simulink model "multipath_fading1"  (Simulink 5.0)
settings: Solver=ode45  StartTime=0.0  StopTime=1  RelTol=1e-3
undefined symbols (not defined in the file): get, p, y
libraries: dspmathops x40, dspstat3 x1, simulink x1, dspsnks4 x1
(part 1 of 2)
settings Model: LastModifiedBy=Daiming Qu  LimitDataPoints=off  SignalLoggingName=logsout  RTWOptions="-aEnforceIntegerDowncast=1 -aExtMode=0 -aExtModeTesting=0 -aFoldNonRolledExpr=1 -aForceParamTrailComments=0 -aGenerateComments=1 -aGenerateReport=0 -aIgnoreCustomStorageClasses=1 -aIncDataTypeInIds=0 -aIncHierarchyInIds=0 -aInlineInvariantSignals=0 -aInlinedPrmAccess=\"Literals\" -aLocalBlockOutputs=1 -aLogVarNameModifier=\"rt_\" -aMaxRTWIdLen=31 -aPrefixModelToSubsysFcnNames=1 -aRTWVerbose=1 -aRollThreshold=5 -aShowEliminatedStatements=0"

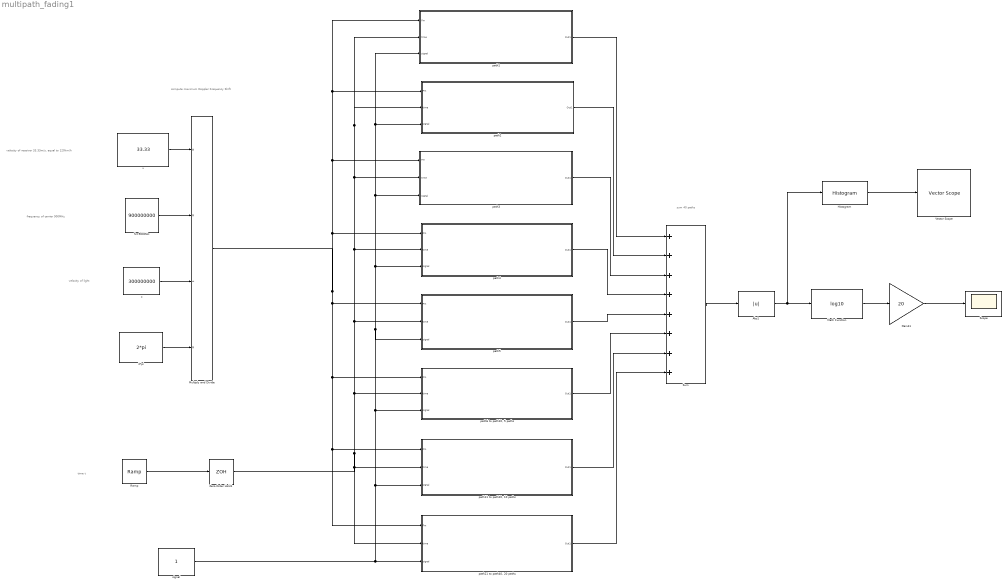
== system multipath_fading1 ==
  note: compute maximum
      | Doppler Frequency Shift
  note: velocity
      |  of light
  note: frequency of carrier
      |  900MHz
  note: velocity of receiver
      | 33.33m/s,
      | equal to 120km/h
  note: sum 40 paths
  note: time t
  2*pi : Constant  Value=2*pi
  Abs1 : Abs
  Gain41 : Gain  Gain=20
  Histogram : dspstat3/Histogram  umin=0  umax=20  nbins=1000  normalized=off  run=on  reset=off  trigtype=Non-zero sample
  Math Function : Math  Operator=log10
  Multiply and Divide : Product  Inputs=**/*  OutScaling=2^-10
  Ramp : simulink/Sources/Ramp  slope=1  start=0  X0=0
  Scope : Scope
      settings: TimeRange=0.06705882352941177  YMax=11  SaveName=ScopeData4
  Sum : Sum  Inputs=++++++++  OutScaling=2^-10
  Vector Scope : dspsnks4/Vector Scope  ScopeProperties=off  Domain=User-defined  HorizSpan=1  DisplayProperties=off  AxisGrid=on  Memory=off  FrameNumber=on  AxisLegend=off  AxisZoom=off  OpenScopeAtSimStart=on  OpenScopeImmediately=off  FigPos=get(0,'defaultfigureposition')  AxisProperties=on  XUnits=Hertz  XRange=[0...Fs/2]  InheritXIncr=on  XIncr=1  XLabel=y  YUnits=dB  YLabel=p(y)  LineProperties=off  LineColors=[0 0 0]
      settings: YMin=0  YMax=700
  Zero-Order Hold1 : ZeroOrderHold  SampleTime=0.00001
  c : Constant  Value=300000000
  fc=900MHz : Constant  Value=900000000
  path1 : Subsystem
  "path11 to path20, 10 paths" : Subsystem
  path2 : Subsystem
  "path21 to path40, 20 paths" : Subsystem
  path3 : Subsystem
  path4 : Subsystem
  path5 : Subsystem
  "path6 to path10, 5 paths" : Subsystem
  signal : Constant
  v : Constant  Value=33.33
  wires:
  fc=900MHz/1 -> Multiply and Divide/2
  c/1 -> Multiply and Divide/3
  v/1 -> Multiply and Divide/1
  Math Function/1 -> Gain41/1
  2*pi/1 -> Multiply and Divide/4
  Gain41/1 -> Scope/1
  Multiply and Divide/1 -> path1/1(Fm), path2/1(Fm), path3/1(Fm), path4/1(Fm), "path6 to path10, 5 paths"/1(Fm), "path21 to path40, 20 paths"/1(Fm), "path11 to path20, 10 paths"/1(Fm), path5/1(Fm)
  path1/1(Out1) -> Sum/1
  "path21 to path40, 20 paths"/1(Out1) -> Sum/8
  "path11 to path20, 10 paths"/1(Out1) -> Sum/7
  "path6 to path10, 5 paths"/1(Out1) -> Sum/6
  Ramp/1 -> Zero-Order Hold1/1
  Zero-Order Hold1/1 -> "path6 to path10, 5 paths"/2(time), path1/2(time), path2/2(time), path3/2(time), path4/2(time), path5/2(time), "path21 to path40, 20 paths"/2(time), "path11 to path20, 10 paths"/2(time)
  Histogram/1 -> Vector Scope/1
  Sum/1 -> Abs1/1
  Abs1/1 -> Histogram/1, Math Function/1
  path2/1(Out1) -> Sum/2
  path3/1(Out1) -> Sum/3
  path4/1(Out1) -> Sum/4
  path5/1(Out1) -> Sum/5
  signal/1 -> "path21 to path40, 20 paths"/3(signal), "path11 to path20, 10 paths"/3(signal), "path6 to path10, 5 paths"/3(signal), path5/3(signal), path4/3(signal), path3/3(signal), path2/3(signal), path1/3(signal)

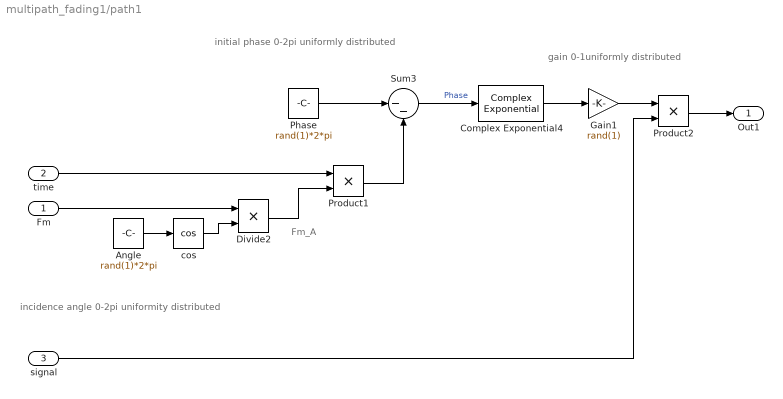
== system multipath_fading1/path1 ==
  note: initial phase
      | 0-2pi
      | uniformly
      | distributed
  note: incidence angle
      | 0-2pi
      | uniformity
      | distributed
  note: gain
      | 0-1uniformly distributed
  note: Fm_A
  Fm : Inport
  time : Inport  Port=2
  signal : Inport  Port=3
  Angle : Constant  Value=rand(1)*2*pi
  Complex Exponential4 : dspmathops/Complex Exponential
  Divide2 : Product  Inputs=**  OutScaling=2^-10
  Gain1 : Gain  Gain=rand(1)
  Phase : Constant  Value=rand(1)*2*pi
  Product1 : Product  RndMeth=Zero
  Product2 : Product  RndMeth=Zero
  Sum3 : Sum  Inputs=|--
  cos : Trigonometry  Operator=cos
  Out1 : Outport
  wires:
  Phase/1 -> Sum3/1
  Complex Exponential4/1 -> Gain1/1
  Sum3/1 -> Complex Exponential4/1  "Phase"
  Angle/1 -> cos/1
  Fm/1 -> Divide2/1
  cos/1 -> Divide2/2
  time/1 -> Product1/1
  Divide2/1 -> Product1/2
  Product1/1 -> Sum3/2
  Gain1/1 -> Product2/1
  Product2/1 -> Out1/1
  signal/1 -> Product2/2

== system multipath_fading1/path11 to path20, 10 paths ==
  Fm : Inport
  time : Inport  Port=2
  signal : Inport  Port=3
  Add : Sum  OutScaling=2^-10
  "path11 to path15, 5 paths" : Subsystem
  "path16 to path20, 5 paths" : Subsystem
  Out1 : Outport
  wires:
  Add/1 -> Out1/1
  Fm/1 -> "path11 to path15, 5 paths"/1(Fm), "path16 to path20, 5 paths"/1(Fm)
  "path11 to path15, 5 paths"/1(Out1) -> Add/1
  time/1 -> "path11 to path15, 5 paths"/2(Time), "path16 to path20, 5 paths"/2(Time)
  "path16 to path20, 5 paths"/1(Out1) -> Add/2
  signal/1 -> "path11 to path15, 5 paths"/3(signal), "path16 to path20, 5 paths"/3(signal)

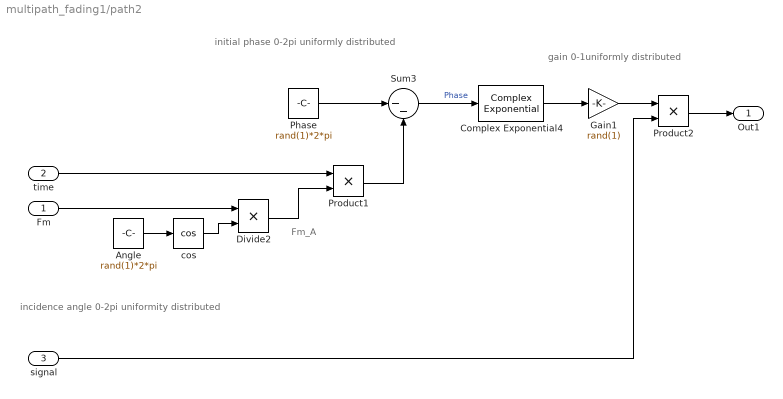
== system multipath_fading1/path2 ==
  note: initial phase
      | 0-2pi
      | uniformly
      | distributed
  note: incidence angle
      | 0-2pi
      | uniformity
      | distributed
  note: gain
      | 0-1uniformly distributed
  note: Fm_A
  Fm : Inport
  time : Inport  Port=2
  signal : Inport  Port=3
  Angle : Constant  Value=rand(1)*2*pi
  Complex Exponential4 : dspmathops/Complex Exponential
  Divide2 : Product  Inputs=**  OutScaling=2^-10
  Gain1 : Gain  Gain=rand(1)
  Phase : Constant  Value=rand(1)*2*pi
  Product1 : Product  RndMeth=Zero
  Product2 : Product  RndMeth=Zero
  Sum3 : Sum  Inputs=|--
  cos : Trigonometry  Operator=cos
  Out1 : Outport
  wires:
  Phase/1 -> Sum3/1
  Complex Exponential4/1 -> Gain1/1
  Sum3/1 -> Complex Exponential4/1  "Phase"
  Angle/1 -> cos/1
  Fm/1 -> Divide2/1
  cos/1 -> Divide2/2
  time/1 -> Product1/1
  Divide2/1 -> Product1/2
  Product1/1 -> Sum3/2
  Gain1/1 -> Product2/1
  Product2/1 -> Out1/1
  signal/1 -> Product2/2

== system multipath_fading1/path21 to path40, 20 paths ==
  Fm : Inport
  time : Inport  Port=2
  signal : Inport  Port=3
  Add : Sum  OutScaling=2^-10
  "path21 to path30, 10 paths" : Subsystem
  "path31 to path40, 10 paths" : Subsystem
  Out1 : Outport
  wires:
  "path31 to path40, 10 paths"/1(Out1) -> Add/2
  time/1 -> "path21 to path30, 10 paths"/2(time), "path31 to path40, 10 paths"/2(time)
  "path21 to path30, 10 paths"/1(Out1) -> Add/1
  Fm/1 -> "path21 to path30, 10 paths"/1(Fm), "path31 to path40, 10 paths"/1(Fm)
  Add/1 -> Out1/1
  signal/1 -> "path21 to path30, 10 paths"/3(signal), "path31 to path40, 10 paths"/3(signal)

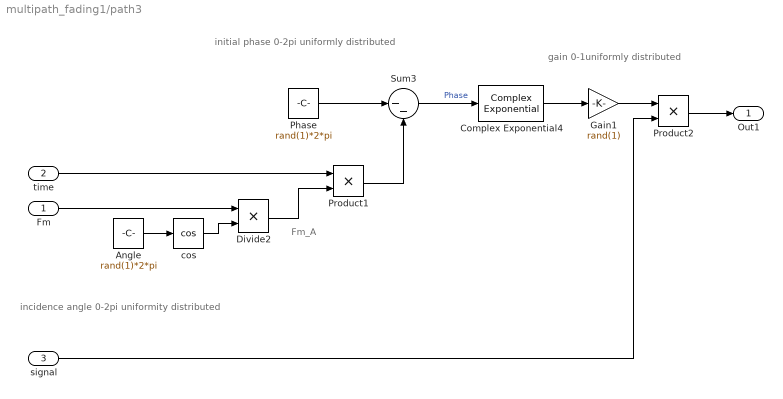
== system multipath_fading1/path3 ==
  note: initial phase
      | 0-2pi
      | uniformly
      | distributed
  note: incidence angle
      | 0-2pi
      | uniformity
      | distributed
  note: gain
      | 0-1uniformly distributed
  note: Fm_A
  Fm : Inport
  time : Inport  Port=2
  signal : Inport  Port=3
  Angle : Constant  Value=rand(1)*2*pi
  Complex Exponential4 : dspmathops/Complex Exponential
  Divide2 : Product  Inputs=**  OutScaling=2^-10
  Gain1 : Gain  Gain=rand(1)
  Phase : Constant  Value=rand(1)*2*pi
  Product1 : Product  RndMeth=Zero
  Product2 : Product  RndMeth=Zero
  Sum3 : Sum  Inputs=|--
  cos : Trigonometry  Operator=cos
  Out1 : Outport
  wires:
  Phase/1 -> Sum3/1
  Complex Exponential4/1 -> Gain1/1
  Sum3/1 -> Complex Exponential4/1  "Phase"
  Angle/1 -> cos/1
  Fm/1 -> Divide2/1
  cos/1 -> Divide2/2
  time/1 -> Product1/1
  Divide2/1 -> Product1/2
  Product1/1 -> Sum3/2
  Gain1/1 -> Product2/1
  Product2/1 -> Out1/1
  signal/1 -> Product2/2

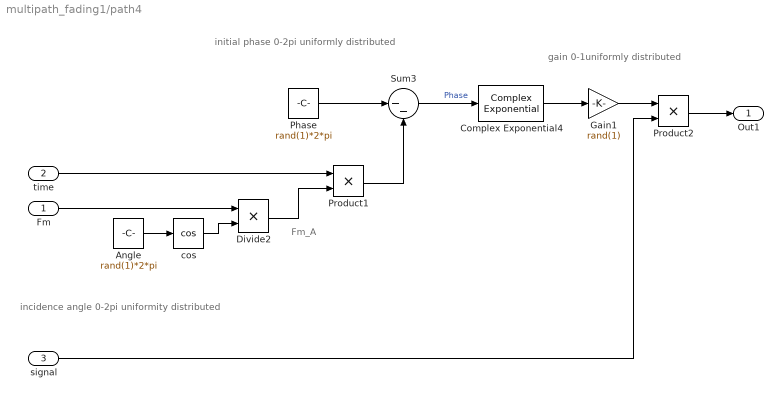
== system multipath_fading1/path4 ==
  note: initial phase
      | 0-2pi
      | uniformly
      | distributed
  note: incidence angle
      | 0-2pi
      | uniformity
      | distributed
  note: gain
      | 0-1uniformly distributed
  note: Fm_A
  Fm : Inport
  time : Inport  Port=2
  signal : Inport  Port=3
  Angle : Constant  Value=rand(1)*2*pi
  Complex Exponential4 : dspmathops/Complex Exponential
  Divide2 : Product  Inputs=**  OutScaling=2^-10
  Gain1 : Gain  Gain=rand(1)
  Phase : Constant  Value=rand(1)*2*pi
  Product1 : Product  RndMeth=Zero
  Product2 : Product  RndMeth=Zero
  Sum3 : Sum  Inputs=|--
  cos : Trigonometry  Operator=cos
  Out1 : Outport
  wires:
  Phase/1 -> Sum3/1
  Complex Exponential4/1 -> Gain1/1
  Sum3/1 -> Complex Exponential4/1  "Phase"
  Angle/1 -> cos/1
  Fm/1 -> Divide2/1
  cos/1 -> Divide2/2
  time/1 -> Product1/1
  Divide2/1 -> Product1/2
  Product1/1 -> Sum3/2
  Gain1/1 -> Product2/1
  Product2/1 -> Out1/1
  signal/1 -> Product2/2

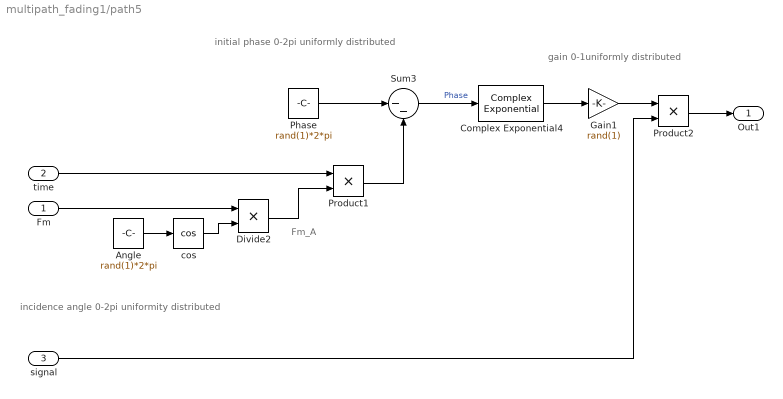
== system multipath_fading1/path5 ==
  note: initial phase
      | 0-2pi
      | uniformly
      | distributed
  note: incidence angle
      | 0-2pi
      | uniformity
      | distributed
  note: gain
      | 0-1uniformly distributed
  note: Fm_A
  Fm : Inport
  time : Inport  Port=2
  signal : Inport  Port=3
  Angle : Constant  Value=rand(1)*2*pi
  Complex Exponential4 : dspmathops/Complex Exponential
  Divide2 : Product  Inputs=**  OutScaling=2^-10
  Gain1 : Gain  Gain=rand(1)
  Phase : Constant  Value=rand(1)*2*pi
  Product1 : Product  RndMeth=Zero
  Product2 : Product  RndMeth=Zero
  Sum3 : Sum  Inputs=|--
  cos : Trigonometry  Operator=cos
  Out1 : Outport
  wires:
  Phase/1 -> Sum3/1
  Complex Exponential4/1 -> Gain1/1
  Sum3/1 -> Complex Exponential4/1  "Phase"
  Angle/1 -> cos/1
  Fm/1 -> Divide2/1
  cos/1 -> Divide2/2
  time/1 -> Product1/1
  Divide2/1 -> Product1/2
  Product1/1 -> Sum3/2
  Gain1/1 -> Product2/1
  Product2/1 -> Out1/1
  signal/1 -> Product2/2

== system multipath_fading1/path6 to path10, 5 paths ==
  Fm : Inport
  time : Inport  Port=2
  signal : Inport  Port=3
  Add : Sum  Inputs=+++++  OutScaling=2^-10
  path1 : Subsystem
  path6 : Subsystem
  path7 : Subsystem
  path8 : Subsystem
  path9 : Subsystem
  Out1 : Outport
  wires:
  Fm/1 -> path9/1(Fm), path1/1(Fm), path8/1(Fm), path7/1(Fm), path6/1(Fm)
  time/1 -> path6/2(time), path7/2(time), path8/2(time), path9/2(time), path1/2(time)
  Add/1 -> Out1/1
  path8/1(Out1) -> Add/3
  path9/1(Out1) -> Add/4
  path7/1(Out1) -> Add/2
  path6/1(Out1) -> Add/1
  path1/1(Out1) -> Add/5
  signal/1 -> path6/3(signal), path7/3(signal), path8/3(signal), path9/3(signal), path1/3(signal)

== system multipath_fading1/path11 to path20, 10 paths/path11 to path15, 5 paths ==
  Fm : Inport
  Time : Inport  Port=2
  signal : Inport  Port=3
  Add : Sum  Inputs=+++++  OutScaling=2^-10
  path11 : Subsystem
  path12 : Subsystem
  path13 : Subsystem
  path14 : Subsystem
  path15 : Subsystem
  Out1 : Outport
  wires:
  Fm/1 -> path14/1(Fm), path15/1(Fm), path13/1(Fm), path12/1(Fm), path11/1(Fm)
  Time/1 -> path11/2(time), path12/2(time), path13/2(time), path14/2(time), path15/2(time)
  Add/1 -> Out1/1
  path13/1(Out1) -> Add/3
  path14/1(Out1) -> Add/4
  path12/1(Out1) -> Add/2
  path11/1(Out1) -> Add/1
  path15/1(Out1) -> Add/5
  signal/1 -> path11/3(signal), path12/3(signal), path13/3(signal), path14/3(signal), path15/3(signal)

== system multipath_fading1/path11 to path20, 10 paths/path16 to path20, 5 paths ==
  Fm : Inport
  Time : Inport  Port=2
  signal : Inport  Port=3
  Add : Sum  Inputs=+++++  OutScaling=2^-10
  path16 : Subsystem
  path17 : Subsystem
  path18 : Subsystem
  path19 : Subsystem
  path20 : Subsystem
  Out1 : Outport
  wires:
  Fm/1 -> path19/1(Fm), path20/1(Fm), path18/1(Fm), path17/1(Fm), path16/1(Fm)
  Time/1 -> path16/2(time), path17/2(time), path18/2(time), path19/2(time), path20/2(time)
  Add/1 -> Out1/1
  path18/1(Out1) -> Add/3
  path19/1(Out1) -> Add/4
  path17/1(Out1) -> Add/2
  path16/1(Out1) -> Add/1
  path20/1(Out1) -> Add/5
  signal/1 -> path16/3(signal), path17/3(signal), path18/3(signal), path19/3(signal), path20/3(signal)

== system multipath_fading1/path21 to path40, 20 paths/path21 to path30, 10 paths ==
  Fm : Inport
  time : Inport  Port=2
  signal : Inport  Port=3
  Add : Sum  OutScaling=2^-10
  "path21 to path25, 5 paths" : Subsystem
  "path26 to path30, 5 paths" : Subsystem
  Out1 : Outport
  wires:
  Add/1 -> Out1/1
  Fm/1 -> "path21 to path25, 5 paths"/1(Fm), "path26 to path30, 5 paths"/1(Fm)
  "path21 to path25, 5 paths"/1(Out1) -> Add/1
  time/1 -> "path21 to path25, 5 paths"/2(Time), "path26 to path30, 5 paths"/2(Time)
  "path26 to path30, 5 paths"/1(Out1) -> Add/2
  signal/1 -> "path21 to path25, 5 paths"/3(signal), "path26 to path30, 5 paths"/3(signal)

== system multipath_fading1/path21 to path40, 20 paths/path31 to path40, 10 paths ==
  Fm : Inport
  time : Inport  Port=2
  signal : Inport  Port=3
  Add : Sum  OutScaling=2^-10
  "path31 to path35, 5 paths" : Subsystem
  "path36 to path40, 5 paths" : Subsystem
  Out1 : Outport
  wires:
  Add/1 -> Out1/1
  Fm/1 -> "path31 to path35, 5 paths"/1(Fm), "path36 to path40, 5 paths"/1(Fm)
  "path31 to path35, 5 paths"/1(Out1) -> Add/1
  time/1 -> "path31 to path35, 5 paths"/2(Time), "path36 to path40, 5 paths"/2(Time)
  "path36 to path40, 5 paths"/1(Out1) -> Add/2
  signal/1 -> "path31 to path35, 5 paths"/3(signal), "path36 to path40, 5 paths"/3(signal)

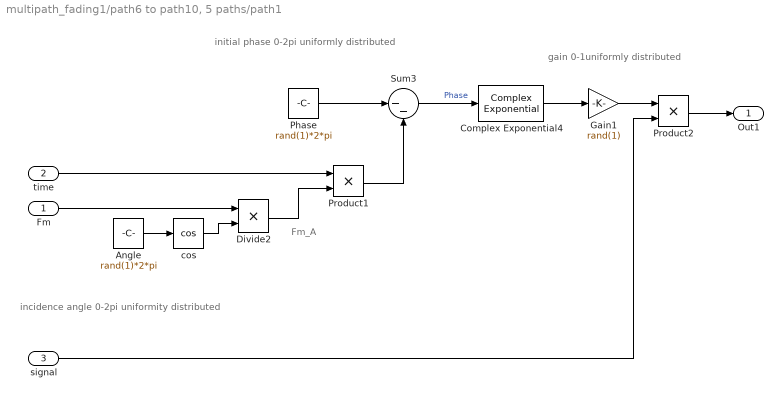
== system multipath_fading1/path6 to path10, 5 paths/path1 ==
  note: initial phase
      | 0-2pi
      | uniformly
      | distributed
  note: incidence angle
      | 0-2pi
      | uniformity
      | distributed
  note: gain
      | 0-1uniformly distributed
  note: Fm_A
  Fm : Inport
  time : Inport  Port=2
  signal : Inport  Port=3
  Angle : Constant  Value=rand(1)*2*pi
  Complex Exponential4 : dspmathops/Complex Exponential
  Divide2 : Product  Inputs=**  OutScaling=2^-10
  Gain1 : Gain  Gain=rand(1)
  Phase : Constant  Value=rand(1)*2*pi
  Product1 : Product  RndMeth=Zero
  Product2 : Product  RndMeth=Zero
  Sum3 : Sum  Inputs=|--
  cos : Trigonometry  Operator=cos
  Out1 : Outport
  wires:
  Phase/1 -> Sum3/1
  Complex Exponential4/1 -> Gain1/1
  Sum3/1 -> Complex Exponential4/1  "Phase"
  Angle/1 -> cos/1
  Fm/1 -> Divide2/1
  cos/1 -> Divide2/2
  time/1 -> Product1/1
  Divide2/1 -> Product1/2
  Product1/1 -> Sum3/2
  Gain1/1 -> Product2/1
  Product2/1 -> Out1/1
  signal/1 -> Product2/2

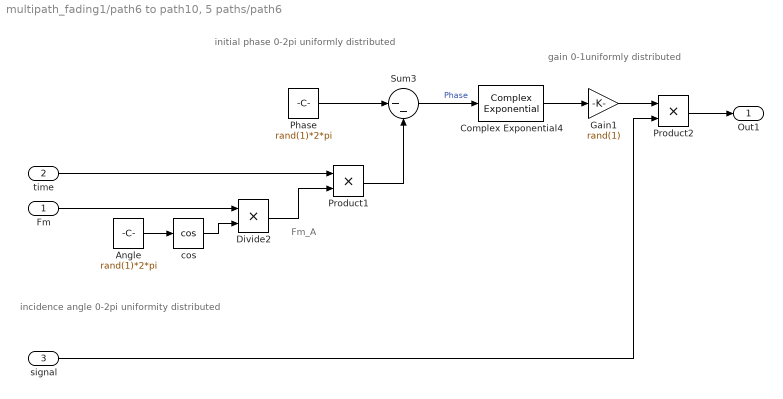
== system multipath_fading1/path6 to path10, 5 paths/path6 ==
  note: initial phase
      | 0-2pi
      | uniformly
      | distributed
  note: incidence angle
      | 0-2pi
      | uniformity
      | distributed
  note: gain
      | 0-1uniformly distributed
  note: Fm_A
  Fm : Inport
  time : Inport  Port=2
  signal : Inport  Port=3
  Angle : Constant  Value=rand(1)*2*pi
  Complex Exponential4 : dspmathops/Complex Exponential
  Divide2 : Product  Inputs=**  OutScaling=2^-10
  Gain1 : Gain  Gain=rand(1)
  Phase : Constant  Value=rand(1)*2*pi
  Product1 : Product  RndMeth=Zero
  Product2 : Product  RndMeth=Zero
  Sum3 : Sum  Inputs=|--
  cos : Trigonometry  Operator=cos
  Out1 : Outport
  wires:
  Phase/1 -> Sum3/1
  Complex Exponential4/1 -> Gain1/1
  Sum3/1 -> Complex Exponential4/1  "Phase"
  Angle/1 -> cos/1
  Fm/1 -> Divide2/1
  cos/1 -> Divide2/2
  time/1 -> Product1/1
  Divide2/1 -> Product1/2
  Product1/1 -> Sum3/2
  Gain1/1 -> Product2/1
  Product2/1 -> Out1/1
  signal/1 -> Product2/2

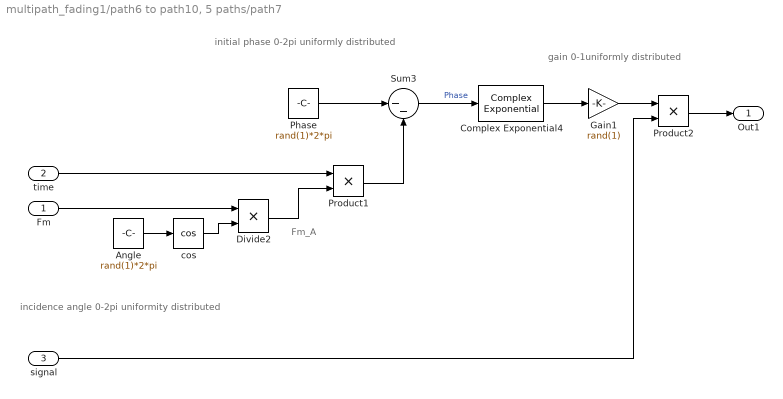
== system multipath_fading1/path6 to path10, 5 paths/path7 ==
  note: initial phase
      | 0-2pi
      | uniformly
      | distributed
  note: incidence angle
      | 0-2pi
      | uniformity
      | distributed
  note: gain
      | 0-1uniformly distributed
  note: Fm_A
  Fm : Inport
  time : Inport  Port=2
  signal : Inport  Port=3
  Angle : Constant  Value=rand(1)*2*pi
  Complex Exponential4 : dspmathops/Complex Exponential
  Divide2 : Product  Inputs=**  OutScaling=2^-10
  Gain1 : Gain  Gain=rand(1)
  Phase : Constant  Value=rand(1)*2*pi
  Product1 : Product  RndMeth=Zero
  Product2 : Product  RndMeth=Zero
  Sum3 : Sum  Inputs=|--
  cos : Trigonometry  Operator=cos
  Out1 : Outport
  wires:
  Phase/1 -> Sum3/1
  Complex Exponential4/1 -> Gain1/1
  Sum3/1 -> Complex Exponential4/1  "Phase"
  Angle/1 -> cos/1
  Fm/1 -> Divide2/1
  cos/1 -> Divide2/2
  time/1 -> Product1/1
  Divide2/1 -> Product1/2
  Product1/1 -> Sum3/2
  Gain1/1 -> Product2/1
  Product2/1 -> Out1/1
  signal/1 -> Product2/2

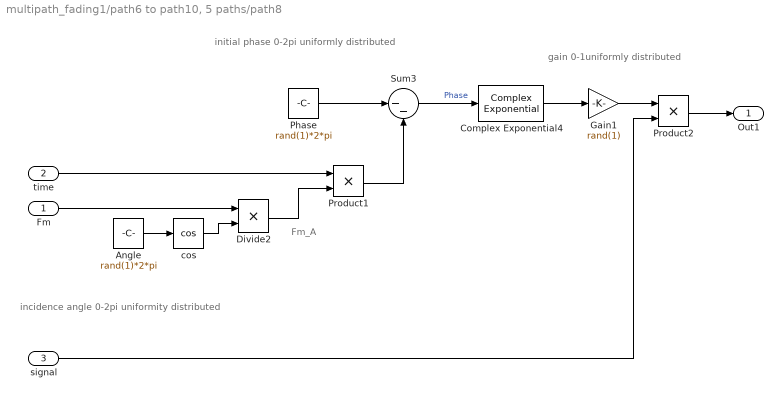
== system multipath_fading1/path6 to path10, 5 paths/path8 ==
  note: initial phase
      | 0-2pi
      | uniformly
      | distributed
  note: incidence angle
      | 0-2pi
      | uniformity
      | distributed
  note: gain
      | 0-1uniformly distributed
  note: Fm_A
  Fm : Inport
  time : Inport  Port=2
  signal : Inport  Port=3
  Angle : Constant  Value=rand(1)*2*pi
  Complex Exponential4 : dspmathops/Complex Exponential
  Divide2 : Product  Inputs=**  OutScaling=2^-10
  Gain1 : Gain  Gain=rand(1)
  Phase : Constant  Value=rand(1)*2*pi
  Product1 : Product  RndMeth=Zero
  Product2 : Product  RndMeth=Zero
  Sum3 : Sum  Inputs=|--
  cos : Trigonometry  Operator=cos
  Out1 : Outport
  wires:
  Phase/1 -> Sum3/1
  Complex Exponential4/1 -> Gain1/1
  Sum3/1 -> Complex Exponential4/1  "Phase"
  Angle/1 -> cos/1
  Fm/1 -> Divide2/1
  cos/1 -> Divide2/2
  time/1 -> Product1/1
  Divide2/1 -> Product1/2
  Product1/1 -> Sum3/2
  Gain1/1 -> Product2/1
  Product2/1 -> Out1/1
  signal/1 -> Product2/2

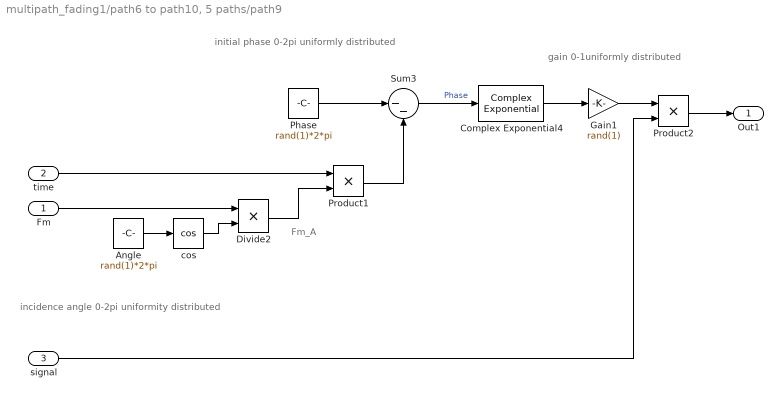
== system multipath_fading1/path6 to path10, 5 paths/path9 ==
  note: initial phase
      | 0-2pi
      | uniformly
      | distributed
  note: incidence angle
      | 0-2pi
      | uniformity
      | distributed
  note: gain
      | 0-1uniformly distributed
  note: Fm_A
  Fm : Inport
  time : Inport  Port=2
  signal : Inport  Port=3
  Angle : Constant  Value=rand(1)*2*pi
  Complex Exponential4 : dspmathops/Complex Exponential
  Divide2 : Product  Inputs=**  OutScaling=2^-10
  Gain1 : Gain  Gain=rand(1)
  Phase : Constant  Value=rand(1)*2*pi
  Product1 : Product  RndMeth=Zero
  Product2 : Product  RndMeth=Zero
  Sum3 : Sum  Inputs=|--
  cos : Trigonometry  Operator=cos
  Out1 : Outport
  wires:
  Phase/1 -> Sum3/1
  Complex Exponential4/1 -> Gain1/1
  Sum3/1 -> Complex Exponential4/1  "Phase"
  Angle/1 -> cos/1
  Fm/1 -> Divide2/1
  cos/1 -> Divide2/2
  time/1 -> Product1/1
  Divide2/1 -> Product1/2
  Product1/1 -> Sum3/2
  Gain1/1 -> Product2/1
  Product2/1 -> Out1/1
  signal/1 -> Product2/2

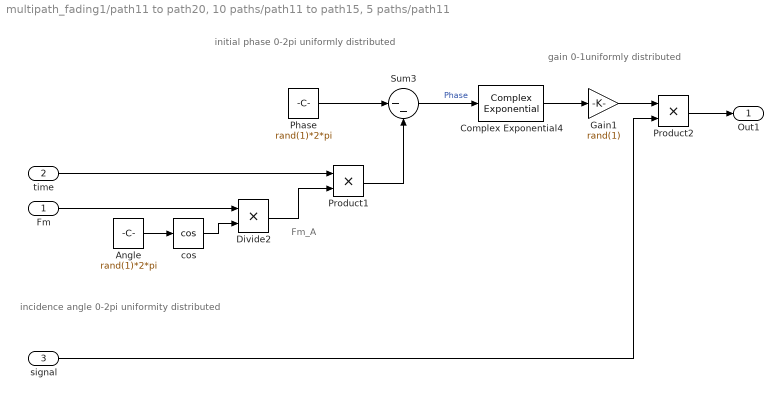
== system multipath_fading1/path11 to path20, 10 paths/path11 to path15, 5 paths/path11 ==
  note: initial phase
      | 0-2pi
      | uniformly
      | distributed
  note: incidence angle
      | 0-2pi
      | uniformity
      | distributed
  note: gain
      | 0-1uniformly distributed
  note: Fm_A
  Fm : Inport
  time : Inport  Port=2
  signal : Inport  Port=3
  Angle : Constant  Value=rand(1)*2*pi
  Complex Exponential4 : dspmathops/Complex Exponential
  Divide2 : Product  Inputs=**  OutScaling=2^-10
  Gain1 : Gain  Gain=rand(1)
  Phase : Constant  Value=rand(1)*2*pi
  Product1 : Product  RndMeth=Zero
  Product2 : Product  RndMeth=Zero
  Sum3 : Sum  Inputs=|--
  cos : Trigonometry  Operator=cos
  Out1 : Outport
  wires:
  Phase/1 -> Sum3/1
  Complex Exponential4/1 -> Gain1/1
  Sum3/1 -> Complex Exponential4/1  "Phase"
  Angle/1 -> cos/1
  Fm/1 -> Divide2/1
  cos/1 -> Divide2/2
  time/1 -> Product1/1
  Divide2/1 -> Product1/2
  Product1/1 -> Sum3/2
  Gain1/1 -> Product2/1
  Product2/1 -> Out1/1
  signal/1 -> Product2/2

== system multipath_fading1/path11 to path20, 10 paths/path11 to path15, 5 paths/path12 ==
  note: initial phase
      | 0-2pi
      | uniformly
      | distributed
  note: incidence angle
      | 0-2pi
      | uniformity
      | distributed
  note: gain
      | 0-1uniformly distributed
  note: Fm_A
  Fm : Inport
  time : Inport  Port=2
  signal : Inport  Port=3
  Angle : Constant  Value=rand(1)*2*pi
  Complex Exponential4 : dspmathops/Complex Exponential
  Divide2 : Product  Inputs=**  OutScaling=2^-10
  Gain1 : Gain  Gain=rand(1)
  Phase : Constant  Value=rand(1)*2*pi
  Product1 : Product  RndMeth=Zero
  Product2 : Product  RndMeth=Zero
  Sum3 : Sum  Inputs=|--
  cos : Trigonometry  Operator=cos
  Out1 : Outport
  wires:
  Phase/1 -> Sum3/1
  Complex Exponential4/1 -> Gain1/1
  Sum3/1 -> Complex Exponential4/1  "Phase"
  Angle/1 -> cos/1
  Fm/1 -> Divide2/1
  cos/1 -> Divide2/2
  time/1 -> Product1/1
  Divide2/1 -> Product1/2
  Product1/1 -> Sum3/2
  Gain1/1 -> Product2/1
  Product2/1 -> Out1/1
  signal/1 -> Product2/2

== system multipath_fading1/path11 to path20, 10 paths/path11 to path15, 5 paths/path13 ==
  note: initial phase
      | 0-2pi
      | uniformly
      | distributed
  note: incidence angle
      | 0-2pi
      | uniformity
      | distributed
  note: gain
      | 0-1uniformly distributed
  note: Fm_A
  Fm : Inport
  time : Inport  Port=2
  signal : Inport  Port=3
  Angle : Constant  Value=rand(1)*2*pi
  Complex Exponential4 : dspmathops/Complex Exponential
  Divide2 : Product  Inputs=**  OutScaling=2^-10
  Gain1 : Gain  Gain=rand(1)
  Phase : Constant  Value=rand(1)*2*pi
  Product1 : Product  RndMeth=Zero
  Product2 : Product  RndMeth=Zero
  Sum3 : Sum  Inputs=|--
  cos : Trigonometry  Operator=cos
  Out1 : Outport
  wires:
  Phase/1 -> Sum3/1
  Complex Exponential4/1 -> Gain1/1
  Sum3/1 -> Complex Exponential4/1  "Phase"
  Angle/1 -> cos/1
  Fm/1 -> Divide2/1
  cos/1 -> Divide2/2
  time/1 -> Product1/1
  Divide2/1 -> Product1/2
  Product1/1 -> Sum3/2
  Gain1/1 -> Product2/1
  Product2/1 -> Out1/1
  signal/1 -> Product2/2

== system multipath_fading1/path11 to path20, 10 paths/path11 to path15, 5 paths/path14 ==
  note: initial phase
      | 0-2pi
      | uniformly
      | distributed
  note: incidence angle
      | 0-2pi
      | uniformity
      | distributed
  note: gain
      | 0-1uniformly distributed
  note: Fm_A
  Fm : Inport
  time : Inport  Port=2
  signal : Inport  Port=3
  Angle : Constant  Value=rand(1)*2*pi
  Complex Exponential4 : dspmathops/Complex Exponential
  Divide2 : Product  Inputs=**  OutScaling=2^-10
  Gain1 : Gain  Gain=rand(1)
  Phase : Constant  Value=rand(1)*2*pi
  Product1 : Product  RndMeth=Zero
  Product2 : Product  RndMeth=Zero
  Sum3 : Sum  Inputs=|--
  cos : Trigonometry  Operator=cos
  Out1 : Outport
  wires:
  Phase/1 -> Sum3/1
  Complex Exponential4/1 -> Gain1/1
  Sum3/1 -> Complex Exponential4/1  "Phase"
  Angle/1 -> cos/1
  Fm/1 -> Divide2/1
  cos/1 -> Divide2/2
  time/1 -> Product1/1
  Divide2/1 -> Product1/2
  Product1/1 -> Sum3/2
  Gain1/1 -> Product2/1
  Product2/1 -> Out1/1
  signal/1 -> Product2/2

== system multipath_fading1/path11 to path20, 10 paths/path11 to path15, 5 paths/path15 ==
  note: initial phase
      | 0-2pi
      | uniformly
      | distributed
  note: incidence angle
      | 0-2pi
      | uniformity
      | distributed
  note: gain
      | 0-1uniformly distributed
  note: Fm_A
  Fm : Inport
  time : Inport  Port=2
  signal : Inport  Port=3
  Angle : Constant  Value=rand(1)*2*pi
  Complex Exponential4 : dspmathops/Complex Exponential
  Divide2 : Product  Inputs=**  OutScaling=2^-10
  Gain1 : Gain  Gain=rand(1)
  Phase : Constant  Value=rand(1)*2*pi
  Product1 : Product  RndMeth=Zero
  Product2 : Product  RndMeth=Zero
  Sum3 : Sum  Inputs=|--
  cos : Trigonometry  Operator=cos
  Out1 : Outport
  wires:
  Phase/1 -> Sum3/1
  Complex Exponential4/1 -> Gain1/1
  Sum3/1 -> Complex Exponential4/1  "Phase"
  Angle/1 -> cos/1
  Fm/1 -> Divide2/1
  cos/1 -> Divide2/2
  time/1 -> Product1/1
  Divide2/1 -> Product1/2
  Product1/1 -> Sum3/2
  Gain1/1 -> Product2/1
  Product2/1 -> Out1/1
  signal/1 -> Product2/2

== system multipath_fading1/path11 to path20, 10 paths/path16 to path20, 5 paths/path16 ==
  note: initial phase
      | 0-2pi
      | uniformly
      | distributed
  note: incidence angle
      | 0-2pi
      | uniformity
      | distributed
  note: gain
      | 0-1uniformly distributed
  note: Fm_A
  Fm : Inport
  time : Inport  Port=2
  signal : Inport  Port=3
  Angle : Constant  Value=rand(1)*2*pi
  Complex Exponential4 : dspmathops/Complex Exponential
  Divide2 : Product  Inputs=**  OutScaling=2^-10
  Gain1 : Gain  Gain=rand(1)
  Phase : Constant  Value=rand(1)*2*pi
  Product1 : Product  RndMeth=Zero
  Product2 : Product  RndMeth=Zero
  Sum3 : Sum  Inputs=|--
  cos : Trigonometry  Operator=cos
  Out1 : Outport
  wires:
  Phase/1 -> Sum3/1
  Complex Exponential4/1 -> Gain1/1
  Sum3/1 -> Complex Exponential4/1  "Phase"
  Angle/1 -> cos/1
  Fm/1 -> Divide2/1
  cos/1 -> Divide2/2
  time/1 -> Product1/1
  Divide2/1 -> Product1/2
  Product1/1 -> Sum3/2
  Gain1/1 -> Product2/1
  Product2/1 -> Out1/1
  signal/1 -> Product2/2

== system multipath_fading1/path11 to path20, 10 paths/path16 to path20, 5 paths/path17 ==
  note: initial phase
      | 0-2pi
      | uniformly
      | distributed
  note: incidence angle
      | 0-2pi
      | uniformity
      | distributed
  note: gain
      | 0-1uniformly distributed
  note: Fm_A
  Fm : Inport
  time : Inport  Port=2
  signal : Inport  Port=3
  Angle : Constant  Value=rand(1)*2*pi
  Complex Exponential4 : dspmathops/Complex Exponential
  Divide2 : Product  Inputs=**  OutScaling=2^-10
  Gain1 : Gain  Gain=rand(1)
  Phase : Constant  Value=rand(1)*2*pi
  Product1 : Product  RndMeth=Zero
  Product2 : Product  RndMeth=Zero
  Sum3 : Sum  Inputs=|--
  cos : Trigonometry  Operator=cos
  Out1 : Outport
  wires:
  Phase/1 -> Sum3/1
  Complex Exponential4/1 -> Gain1/1
  Sum3/1 -> Complex Exponential4/1  "Phase"
  Angle/1 -> cos/1
  Fm/1 -> Divide2/1
  cos/1 -> Divide2/2
  time/1 -> Product1/1
  Divide2/1 -> Product1/2
  Product1/1 -> Sum3/2
  Gain1/1 -> Product2/1
  Product2/1 -> Out1/1
  signal/1 -> Product2/2

== system multipath_fading1/path11 to path20, 10 paths/path16 to path20, 5 paths/path18 ==
  note: initial phase
      | 0-2pi
      | uniformly
      | distributed
  note: incidence angle
      | 0-2pi
      | uniformity
      | distributed
  note: gain
      | 0-1uniformly distributed
  note: Fm_A
  Fm : Inport
  time : Inport  Port=2
  signal : Inport  Port=3
  Angle : Constant  Value=rand(1)*2*pi
  Complex Exponential4 : dspmathops/Complex Exponential
  Divide2 : Product  Inputs=**  OutScaling=2^-10
  Gain1 : Gain  Gain=rand(1)
  Phase : Constant  Value=rand(1)*2*pi
  Product1 : Product  RndMeth=Zero
  Product2 : Product  RndMeth=Zero
  Sum3 : Sum  Inputs=|--
  cos : Trigonometry  Operator=cos
  Out1 : Outport
  wires:
  Phase/1 -> Sum3/1
  Complex Exponential4/1 -> Gain1/1
  Sum3/1 -> Complex Exponential4/1  "Phase"
  Angle/1 -> cos/1
  Fm/1 -> Divide2/1
  cos/1 -> Divide2/2
  time/1 -> Product1/1
  Divide2/1 -> Product1/2
  Product1/1 -> Sum3/2
  Gain1/1 -> Product2/1
  Product2/1 -> Out1/1
  signal/1 -> Product2/2

== system multipath_fading1/path11 to path20, 10 paths/path16 to path20, 5 paths/path19 ==
  note: initial phase
      | 0-2pi
      | uniformly
      | distributed
  note: incidence angle
      | 0-2pi
      | uniformity
      | distributed
  note: gain
      | 0-1uniformly distributed
  note: Fm_A
  Fm : Inport
  time : Inport  Port=2
  signal : Inport  Port=3
  Angle : Constant  Value=rand(1)*2*pi
  Complex Exponential4 : dspmathops/Complex Exponential
  Divide2 : Product  Inputs=**  OutScaling=2^-10
  Gain1 : Gain  Gain=rand(1)
  Phase : Constant  Value=rand(1)*2*pi
  Product1 : Product  RndMeth=Zero
  Product2 : Product  RndMeth=Zero
  Sum3 : Sum  Inputs=|--
  cos : Trigonometry  Operator=cos
  Out1 : Outport
  wires:
  Phase/1 -> Sum3/1
  Complex Exponential4/1 -> Gain1/1
  Sum3/1 -> Complex Exponential4/1  "Phase"
  Angle/1 -> cos/1
  Fm/1 -> Divide2/1
  cos/1 -> Divide2/2
  time/1 -> Product1/1
  Divide2/1 -> Product1/2
  Product1/1 -> Sum3/2
  Gain1/1 -> Product2/1
  Product2/1 -> Out1/1
  signal/1 -> Product2/2

== system multipath_fading1/path11 to path20, 10 paths/path16 to path20, 5 paths/path20 ==
  note: initial phase
      | 0-2pi
      | uniformly
      | distributed
  note: incidence angle
      | 0-2pi
      | uniformity
      | distributed
  note: gain
      | 0-1uniformly distributed
  note: Fm_A
  Fm : Inport
  time : Inport  Port=2
  signal : Inport  Port=3
  Angle : Constant  Value=rand(1)*2*pi
  Complex Exponential4 : dspmathops/Complex Exponential
  Divide2 : Product  Inputs=**  OutScaling=2^-10
  Gain1 : Gain  Gain=rand(1)
  Phase : Constant  Value=rand(1)*2*pi
  Product1 : Product  RndMeth=Zero
  Product2 : Product  RndMeth=Zero
  Sum3 : Sum  Inputs=|--
  cos : Trigonometry  Operator=cos
  Out1 : Outport
  wires:
  Phase/1 -> Sum3/1
  Complex Exponential4/1 -> Gain1/1
  Sum3/1 -> Complex Exponential4/1  "Phase"
  Angle/1 -> cos/1
  Fm/1 -> Divide2/1
  cos/1 -> Divide2/2
  time/1 -> Product1/1
  Divide2/1 -> Product1/2
  Product1/1 -> Sum3/2
  Gain1/1 -> Product2/1
  Product2/1 -> Out1/1
  signal/1 -> Product2/2

== system multipath_fading1/path21 to path40, 20 paths/path21 to path30, 10 paths/path21 to path25, 5 paths ==
  Fm : Inport
  Time : Inport  Port=2
  signal : Inport  Port=3
  Add : Sum  Inputs=+++++  OutScaling=2^-10
  path21 : Subsystem
  path22 : Subsystem
  path23 : Subsystem
  path24 : Subsystem
  path25 : Subsystem
  Out1 : Outport
  wires:
  Fm/1 -> path24/1(Fm), path25/1(Fm), path23/1(Fm), path22/1(Fm), path21/1(Fm)
  Time/1 -> path21/2(time), path22/2(time), path23/2(time), path24/2(time), path25/2(time)
  Add/1 -> Out1/1
  path23/1(Out1) -> Add/3
  path24/1(Out1) -> Add/4
  path22/1(Out1) -> Add/2
  path21/1(Out1) -> Add/1
  path25/1(Out1) -> Add/5
  signal/1 -> path21/3(signal), path22/3(signal), path23/3(signal), path24/3(signal), path25/3(signal)

== system multipath_fading1/path21 to path40, 20 paths/path21 to path30, 10 paths/path26 to path30, 5 paths ==
  Fm : Inport
  Time : Inport  Port=2
  signal : Inport  Port=3
  Add : Sum  Inputs=+++++  OutScaling=2^-10
  path26 : Subsystem
  path27 : Subsystem
  path28 : Subsystem
  path29 : Subsystem
  path30 : Subsystem
  Out1 : Outport
  wires:
  Fm/1 -> path29/1(Fm), path30/1(Fm), path28/1(Fm), path27/1(Fm), path26/1(Fm)
  Time/1 -> path26/2(time), path27/2(time), path28/2(time), path29/2(time), path30/2(time)
  Add/1 -> Out1/1
  path28/1(Out1) -> Add/3
  path29/1(Out1) -> Add/4
  path27/1(Out1) -> Add/2
  path26/1(Out1) -> Add/1
  path30/1(Out1) -> Add/5
  signal/1 -> path26/3(signal), path27/3(signal), path28/3(signal), path29/3(signal), path30/3(signal)

== system multipath_fading1/path21 to path40, 20 paths/path31 to path40, 10 paths/path31 to path35, 5 paths ==
  Fm : Inport
  Time : Inport  Port=2
  signal : Inport  Port=3
  Add : Sum  Inputs=+++++  OutScaling=2^-10
  path31 : Subsystem
  path32 : Subsystem
  path33 : Subsystem
  path34 : Subsystem
  path35 : Subsystem
  Out1 : Outport
  wires:
  Fm/1 -> path34/1(Fm), path35/1(Fm), path33/1(Fm), path32/1(Fm), path31/1(Fm)
  Time/1 -> path31/2(time), path32/2(time), path33/2(time), path34/2(time), path35/2(time)
  Add/1 -> Out1/1
  path33/1(Out1) -> Add/3
  path34/1(Out1) -> Add/4
  path32/1(Out1) -> Add/2
  path31/1(Out1) -> Add/1
  path35/1(Out1) -> Add/5
  signal/1 -> path31/3(signal), path32/3(signal), path33/3(signal), path34/3(signal), path35/3(signal)

== system multipath_fading1/path21 to path40, 20 paths/path31 to path40, 10 paths/path36 to path40, 5 paths ==
  Fm : Inport
  Time : Inport  Port=2
  signal : Inport  Port=3
  Add : Sum  Inputs=+++++  OutScaling=2^-10
  path36 : Subsystem
  path37 : Subsystem
  path38 : Subsystem
  path39 : Subsystem
  path40 : Subsystem
  Out1 : Outport
  wires:
  Fm/1 -> path39/1(Fm), path40/1(Fm), path38/1(Fm), path37/1(Fm), path36/1(Fm)
  Time/1 -> path36/2(time), path37/2(time), path38/2(time), path39/2(time), path40/2(time)
  Add/1 -> Out1/1
  path38/1(Out1) -> Add/3
  path39/1(Out1) -> Add/4
  path37/1(Out1) -> Add/2
  path36/1(Out1) -> Add/1
  path40/1(Out1) -> Add/5
  signal/1 -> path36/3(signal), path37/3(signal), path38/3(signal), path39/3(signal), path40/3(signal)

== system multipath_fading1/path21 to path40, 20 paths/path21 to path30, 10 paths/path21 to path25, 5 paths/path21 ==
  note: initial phase
      | 0-2pi
      | uniformly
      | distributed
  note: incidence angle
      | 0-2pi
      | uniformity
      | distributed
  note: gain
      | 0-1uniformly distributed
  note: Fm_A
  Fm : Inport
  time : Inport  Port=2
  signal : Inport  Port=3
  Angle : Constant  Value=rand(1)*2*pi
  Complex Exponential4 : dspmathops/Complex Exponential
  Divide2 : Product  Inputs=**  OutScaling=2^-10
  Gain1 : Gain  Gain=rand(1)
  Phase : Constant  Value=rand(1)*2*pi
  Product1 : Product  RndMeth=Zero
  Product2 : Product  RndMeth=Zero
  Sum3 : Sum  Inputs=|--
  cos : Trigonometry  Operator=cos
  Out1 : Outport
  wires:
  Phase/1 -> Sum3/1
  Complex Exponential4/1 -> Gain1/1
  Sum3/1 -> Complex Exponential4/1  "Phase"
  Angle/1 -> cos/1
  Fm/1 -> Divide2/1
  cos/1 -> Divide2/2
  time/1 -> Product1/1
  Divide2/1 -> Product1/2
  Product1/1 -> Sum3/2
  Gain1/1 -> Product2/1
  Product2/1 -> Out1/1
  signal/1 -> Product2/2

== system multipath_fading1/path21 to path40, 20 paths/path21 to path30, 10 paths/path21 to path25, 5 paths/path22 ==
  note: initial phase
      | 0-2pi
      | uniformly
      | distributed
  note: incidence angle
      | 0-2pi
      | uniformity
      | distributed
  note: gain
      | 0-1uniformly distributed
  note: Fm_A
  Fm : Inport
  time : Inport  Port=2
  signal : Inport  Port=3
  Angle : Constant  Value=rand(1)*2*pi
  Complex Exponential4 : dspmathops/Complex Exponential
  Divide2 : Product  Inputs=**  OutScaling=2^-10
  Gain1 : Gain  Gain=rand(1)
  Phase : Constant  Value=rand(1)*2*pi
  Product1 : Product  RndMeth=Zero
  Product2 : Product  RndMeth=Zero
  Sum3 : Sum  Inputs=|--
  cos : Trigonometry  Operator=cos
  Out1 : Outport
  wires:
  Phase/1 -> Sum3/1
  Complex Exponential4/1 -> Gain1/1
  Sum3/1 -> Complex Exponential4/1  "Phase"
  Angle/1 -> cos/1
  Fm/1 -> Divide2/1
  cos/1 -> Divide2/2
  time/1 -> Product1/1
  Divide2/1 -> Product1/2
  Product1/1 -> Sum3/2
  Gain1/1 -> Product2/1
  Product2/1 -> Out1/1
  signal/1 -> Product2/2

== system multipath_fading1/path21 to path40, 20 paths/path21 to path30, 10 paths/path21 to path25, 5 paths/path23 ==
  note: initial phase
      | 0-2pi
      | uniformly
      | distributed
  note: incidence angle
      | 0-2pi
      | uniformity
      | distributed
  note: gain
      | 0-1uniformly distributed
  note: Fm_A
  Fm : Inport
  time : Inport  Port=2
  signal : Inport  Port=3
  Angle : Constant  Value=rand(1)*2*pi
  Complex Exponential4 : dspmathops/Complex Exponential
  Divide2 : Product  Inputs=**  OutScaling=2^-10
  Gain1 : Gain  Gain=rand(1)
  Phase : Constant  Value=rand(1)*2*pi
  Product1 : Product  RndMeth=Zero
  Product2 : Product  RndMeth=Zero
  Sum3 : Sum  Inputs=|--
  cos : Trigonometry  Operator=cos
  Out1 : Outport
  wires:
  Phase/1 -> Sum3/1
  Complex Exponential4/1 -> Gain1/1
  Sum3/1 -> Complex Exponential4/1  "Phase"
  Angle/1 -> cos/1
  Fm/1 -> Divide2/1
  cos/1 -> Divide2/2
  time/1 -> Product1/1
  Divide2/1 -> Product1/2
  Product1/1 -> Sum3/2
  Gain1/1 -> Product2/1
  Product2/1 -> Out1/1
  signal/1 -> Product2/2

== system multipath_fading1/path21 to path40, 20 paths/path21 to path30, 10 paths/path21 to path25, 5 paths/path24 ==
  note: initial phase
      | 0-2pi
      | uniformly
      | distributed
  note: incidence angle
      | 0-2pi
      | uniformity
      | distributed
  note: gain
      | 0-1uniformly distributed
  note: Fm_A
  Fm : Inport
  time : Inport  Port=2
  signal : Inport  Port=3
  Angle : Constant  Value=rand(1)*2*pi
  Complex Exponential4 : dspmathops/Complex Exponential
  Divide2 : Product  Inputs=**  OutScaling=2^-10
  Gain1 : Gain  Gain=rand(1)
  Phase : Constant  Value=rand(1)*2*pi
  Product1 : Product  RndMeth=Zero
  Product2 : Product  RndMeth=Zero
  Sum3 : Sum  Inputs=|--
  cos : Trigonometry  Operator=cos
  Out1 : Outport
  wires:
  Phase/1 -> Sum3/1
  Complex Exponential4/1 -> Gain1/1
  Sum3/1 -> Complex Exponential4/1  "Phase"
  Angle/1 -> cos/1
  Fm/1 -> Divide2/1
  cos/1 -> Divide2/2
  time/1 -> Product1/1
  Divide2/1 -> Product1/2
  Product1/1 -> Sum3/2
  Gain1/1 -> Product2/1
  Product2/1 -> Out1/1
  signal/1 -> Product2/2

== system multipath_fading1/path21 to path40, 20 paths/path21 to path30, 10 paths/path21 to path25, 5 paths/path25 ==
  note: initial phase
      | 0-2pi
      | uniformly
      | distributed
  note: incidence angle
      | 0-2pi
      | uniformity
      | distributed
  note: gain
      | 0-1uniformly distributed
  note: Fm_A
  Fm : Inport
  time : Inport  Port=2
  signal : Inport  Port=3
  Angle : Constant  Value=rand(1)*2*pi
  Complex Exponential4 : dspmathops/Complex Exponential
  Divide2 : Product  Inputs=**  OutScaling=2^-10
  Gain1 : Gain  Gain=rand(1)
  Phase : Constant  Value=rand(1)*2*pi
  Product1 : Product  RndMeth=Zero
  Product2 : Product  RndMeth=Zero
  Sum3 : Sum  Inputs=|--
  cos : Trigonometry  Operator=cos
  Out1 : Outport
  wires:
  Phase/1 -> Sum3/1
  Complex Exponential4/1 -> Gain1/1
  Sum3/1 -> Complex Exponential4/1  "Phase"
  Angle/1 -> cos/1
  Fm/1 -> Divide2/1
  cos/1 -> Divide2/2
  time/1 -> Product1/1
  Divide2/1 -> Product1/2
  Product1/1 -> Sum3/2
  Gain1/1 -> Product2/1
  Product2/1 -> Out1/1
  signal/1 -> Product2/2

== system multipath_fading1/path21 to path40, 20 paths/path21 to path30, 10 paths/path26 to path30, 5 paths/path26 ==
  note: initial phase
      | 0-2pi
      | uniformly
      | distributed
  note: incidence angle
      | 0-2pi
      | uniformity
      | distributed
  note: gain
      | 0-1uniformly distributed
  note: Fm_A
  Fm : Inport
  time : Inport  Port=2
  signal : Inport  Port=3
  Angle : Constant  Value=rand(1)*2*pi
  Complex Exponential4 : dspmathops/Complex Exponential
  Divide2 : Product  Inputs=**  OutScaling=2^-10
  Gain1 : Gain  Gain=rand(1)
  Phase : Constant  Value=rand(1)*2*pi
  Product1 : Product  RndMeth=Zero
  Product2 : Product  RndMeth=Zero
  Sum3 : Sum  Inputs=|--
  cos : Trigonometry  Operator=cos
  Out1 : Outport
  wires:
  Phase/1 -> Sum3/1
  Complex Exponential4/1 -> Gain1/1
  Sum3/1 -> Complex Exponential4/1  "Phase"
  Angle/1 -> cos/1
  Fm/1 -> Divide2/1
  cos/1 -> Divide2/2
  time/1 -> Product1/1
  Divide2/1 -> Product1/2
  Product1/1 -> Sum3/2
  Gain1/1 -> Product2/1
  Product2/1 -> Out1/1
  signal/1 -> Product2/2

== system multipath_fading1/path21 to path40, 20 paths/path21 to path30, 10 paths/path26 to path30, 5 paths/path27 ==
  note: initial phase
      | 0-2pi
      | uniformly
      | distributed
  note: incidence angle
      | 0-2pi
      | uniformity
      | distributed
  note: gain
      | 0-1uniformly distributed
  note: Fm_A
  Fm : Inport
  time : Inport  Port=2
  signal : Inport  Port=3
  Angle : Constant  Value=rand(1)*2*pi
  Complex Exponential4 : dspmathops/Complex Exponential
  Divide2 : Product  Inputs=**  OutScaling=2^-10
  Gain1 : Gain  Gain=rand(1)
  Phase : Constant  Value=rand(1)*2*pi
  Product1 : Product  RndMeth=Zero
  Product2 : Product  RndMeth=Zero
  Sum3 : Sum  Inputs=|--
  cos : Trigonometry  Operator=cos
  Out1 : Outport
  wires:
  Phase/1 -> Sum3/1
  Complex Exponential4/1 -> Gain1/1
  Sum3/1 -> Complex Exponential4/1  "Phase"
  Angle/1 -> cos/1
  Fm/1 -> Divide2/1
  cos/1 -> Divide2/2
  time/1 -> Product1/1
  Divide2/1 -> Product1/2
  Product1/1 -> Sum3/2
  Gain1/1 -> Product2/1
  Product2/1 -> Out1/1
  signal/1 -> Product2/2

== system multipath_fading1/path21 to path40, 20 paths/path21 to path30, 10 paths/path26 to path30, 5 paths/path28 ==
  note: initial phase
      | 0-2pi
      | uniformly
      | distributed
  note: incidence angle
      | 0-2pi
      | uniformity
      | distributed
  note: gain
      | 0-1uniformly distributed
  note: Fm_A
  Fm : Inport
  time : Inport  Port=2
  signal : Inport  Port=3
  Angle : Constant  Value=rand(1)*2*pi
  Complex Exponential4 : dspmathops/Complex Exponential
  Divide2 : Product  Inputs=**  OutScaling=2^-10
  Gain1 : Gain  Gain=rand(1)
  Phase : Constant  Value=rand(1)*2*pi
  Product1 : Product  RndMeth=Zero
  Product2 : Product  RndMeth=Zero
  Sum3 : Sum  Inputs=|--
  cos : Trigonometry  Operator=cos
  Out1 : Outport
  wires:
  Phase/1 -> Sum3/1
  Complex Exponential4/1 -> Gain1/1
  Sum3/1 -> Complex Exponential4/1  "Phase"
  Angle/1 -> cos/1
  Fm/1 -> Divide2/1
  cos/1 -> Divide2/2
  time/1 -> Product1/1
  Divide2/1 -> Product1/2
  Product1/1 -> Sum3/2
  Gain1/1 -> Product2/1
  Product2/1 -> Out1/1
  signal/1 -> Product2/2

== system multipath_fading1/path21 to path40, 20 paths/path21 to path30, 10 paths/path26 to path30, 5 paths/path29 ==
  note: initial phase
      | 0-2pi
      | uniformly
      | distributed
  note: incidence angle
      | 0-2pi
      | uniformity
      | distributed
  note: gain
      | 0-1uniformly distributed
  note: Fm_A
  Fm : Inport
  time : Inport  Port=2
  signal : Inport  Port=3
  Angle : Constant  Value=rand(1)*2*pi
  Complex Exponential4 : dspmathops/Complex Exponential
  Divide2 : Product  Inputs=**  OutScaling=2^-10
  Gain1 : Gain  Gain=rand(1)
  Phase : Constant  Value=rand(1)*2*pi
  Product1 : Product  RndMeth=Zero
  Product2 : Product  RndMeth=Zero
  Sum3 : Sum  Inputs=|--
  cos : Trigonometry  Operator=cos
  Out1 : Outport
  wires:
  Phase/1 -> Sum3/1
  Complex Exponential4/1 -> Gain1/1
  Sum3/1 -> Complex Exponential4/1  "Phase"
  Angle/1 -> cos/1
  Fm/1 -> Divide2/1
  cos/1 -> Divide2/2
  time/1 -> Product1/1
  Divide2/1 -> Product1/2
  Product1/1 -> Sum3/2
  Gain1/1 -> Product2/1
  Product2/1 -> Out1/1
  signal/1 -> Product2/2

== system multipath_fading1/path21 to path40, 20 paths/path21 to path30, 10 paths/path26 to path30, 5 paths/path30 ==
  note: initial phase
      | 0-2pi
      | uniformly
      | distributed
  note: incidence angle
      | 0-2pi
      | uniformity
      | distributed
  note: gain
      | 0-1uniformly distributed
  note: Fm_A
  Fm : Inport
  time : Inport  Port=2
  signal : Inport  Port=3
  Angle : Constant  Value=rand(1)*2*pi
  Complex Exponential4 : dspmathops/Complex Exponential
  Divide2 : Product  Inputs=**  OutScaling=2^-10
  Gain1 : Gain  Gain=rand(1)
  Phase : Constant  Value=rand(1)*2*pi
  Product1 : Product  RndMeth=Zero
  Product2 : Product  RndMeth=Zero
  Sum3 : Sum  Inputs=|--
  cos : Trigonometry  Operator=cos
  Out1 : Outport
  wires:
  Phase/1 -> Sum3/1
  Complex Exponential4/1 -> Gain1/1
  Sum3/1 -> Complex Exponential4/1  "Phase"
  Angle/1 -> cos/1
  Fm/1 -> Divide2/1
  cos/1 -> Divide2/2
  time/1 -> Product1/1
  Divide2/1 -> Product1/2
  Product1/1 -> Sum3/2
  Gain1/1 -> Product2/1
  Product2/1 -> Out1/1
  signal/1 -> Product2/2

== system multipath_fading1/path21 to path40, 20 paths/path31 to path40, 10 paths/path31 to path35, 5 paths/path31 ==
  note: initial phase
      | 0-2pi
      | uniformly
      | distributed
  note: incidence angle
      | 0-2pi
      | uniformity
      | distributed
  note: gain
      | 0-1uniformly distributed
  note: Fm_A
  Fm : Inport
  time : Inport  Port=2
  signal : Inport  Port=3
  Angle : Constant  Value=rand(1)*2*pi
  Complex Exponential4 : dspmathops/Complex Exponential
  Divide2 : Product  Inputs=**  OutScaling=2^-10
  Gain1 : Gain  Gain=rand(1)
  Phase : Constant  Value=rand(1)*2*pi
  Product1 : Product  RndMeth=Zero
  Product2 : Product  RndMeth=Zero
  Sum3 : Sum  Inputs=|--
  cos : Trigonometry  Operator=cos
  Out1 : Outport
  wires:
  Phase/1 -> Sum3/1
  Complex Exponential4/1 -> Gain1/1
  Sum3/1 -> Complex Exponential4/1  "Phase"
  Angle/1 -> cos/1
  Fm/1 -> Divide2/1
  cos/1 -> Divide2/2
  time/1 -> Product1/1
  Divide2/1 -> Product1/2
  Product1/1 -> Sum3/2
  Gain1/1 -> Product2/1
  Product2/1 -> Out1/1
  signal/1 -> Product2/2

== system multipath_fading1/path21 to path40, 20 paths/path31 to path40, 10 paths/path31 to path35, 5 paths/path32 ==
  note: initial phase
      | 0-2pi
      | uniformly
      | distributed
  note: incidence angle
      | 0-2pi
      | uniformity
      | distributed
  note: gain
      | 0-1uniformly distributed
  note: Fm_A
  Fm : Inport
  time : Inport  Port=2
  signal : Inport  Port=3
  Angle : Constant  Value=rand(1)*2*pi
  Complex Exponential4 : dspmathops/Complex Exponential
  Divide2 : Product  Inputs=**  OutScaling=2^-10
  Gain1 : Gain  Gain=rand(1)
  Phase : Constant  Value=rand(1)*2*pi
  Product1 : Product  RndMeth=Zero
  Product2 : Product  RndMeth=Zero
  Sum3 : Sum  Inputs=|--
  cos : Trigonometry  Operator=cos
  Out1 : Outport
  wires:
  Phase/1 -> Sum3/1
  Complex Exponential4/1 -> Gain1/1
  Sum3/1 -> Complex Exponential4/1  "Phase"
  Angle/1 -> cos/1
  Fm/1 -> Divide2/1
  cos/1 -> Divide2/2
  time/1 -> Product1/1
  Divide2/1 -> Product1/2
  Product1/1 -> Sum3/2
  Gain1/1 -> Product2/1
  Product2/1 -> Out1/1
  signal/1 -> Product2/2

== system multipath_fading1/path21 to path40, 20 paths/path31 to path40, 10 paths/path31 to path35, 5 paths/path33 ==
  note: initial phase
      | 0-2pi
      | uniformly
      | distributed
  note: incidence angle
      | 0-2pi
      | uniformity
      | distributed
  note: gain
      | 0-1uniformly distributed
  note: Fm_A
  Fm : Inport
  time : Inport  Port=2
  signal : Inport  Port=3
  Angle : Constant  Value=rand(1)*2*pi
  Complex Exponential4 : dspmathops/Complex Exponential
  Divide2 : Product  Inputs=**  OutScaling=2^-10
  Gain1 : Gain  Gain=rand(1)
  Phase : Constant  Value=rand(1)*2*pi
  Product1 : Product  RndMeth=Zero
  Product2 : Product  RndMeth=Zero
  Sum3 : Sum  Inputs=|--
  cos : Trigonometry  Operator=cos
  Out1 : Outport
  wires:
  Phase/1 -> Sum3/1
  Complex Exponential4/1 -> Gain1/1
  Sum3/1 -> Complex Exponential4/1  "Phase"
  Angle/1 -> cos/1
  Fm/1 -> Divide2/1
  cos/1 -> Divide2/2
  time/1 -> Product1/1
  Divide2/1 -> Product1/2
  Product1/1 -> Sum3/2
  Gain1/1 -> Product2/1
  Product2/1 -> Out1/1
  signal/1 -> Product2/2

== system multipath_fading1/path21 to path40, 20 paths/path31 to path40, 10 paths/path31 to path35, 5 paths/path34 ==
  note: initial phase
      | 0-2pi
      | uniformly
      | distributed
  note: incidence angle
      | 0-2pi
      | uniformity
      | distributed
  note: gain
      | 0-1uniformly distributed
  note: Fm_A
  Fm : Inport
  time : Inport  Port=2
  signal : Inport  Port=3
  Angle : Constant  Value=rand(1)*2*pi
  Complex Exponential4 : dspmathops/Complex Exponential
  Divide2 : Product  Inputs=**  OutScaling=2^-10
  Gain1 : Gain  Gain=rand(1)
  Phase : Constant  Value=rand(1)*2*pi
  Product1 : Product  RndMeth=Zero
  Product2 : Product  RndMeth=Zero
  Sum3 : Sum  Inputs=|--
  cos : Trigonometry  Operator=cos
  Out1 : Outport
  wires:
  Phase/1 -> Sum3/1
  Complex Exponential4/1 -> Gain1/1
  Sum3/1 -> Complex Exponential4/1  "Phase"
  Angle/1 -> cos/1
  Fm/1 -> Divide2/1
  cos/1 -> Divide2/2
  time/1 -> Product1/1
  Divide2/1 -> Product1/2
  Product1/1 -> Sum3/2
  Gain1/1 -> Product2/1
  Product2/1 -> Out1/1
  signal/1 -> Product2/2

== system multipath_fading1/path21 to path40, 20 paths/path31 to path40, 10 paths/path31 to path35, 5 paths/path35 ==
  note: initial phase
      | 0-2pi
      | uniformly
      | distributed
  note: incidence angle
      | 0-2pi
      | uniformity
      | distributed
  note: gain
      | 0-1uniformly distributed
  note: Fm_A
  Fm : Inport
  time : Inport  Port=2
  signal : Inport  Port=3
  Angle : Constant  Value=rand(1)*2*pi
  Complex Exponential4 : dspmathops/Complex Exponential
  Divide2 : Product  Inputs=**  OutScaling=2^-10
  Gain1 : Gain  Gain=rand(1)
  Phase : Constant  Value=rand(1)*2*pi
  Product1 : Product  RndMeth=Zero
  Product2 : Product  RndMeth=Zero
  Sum3 : Sum  Inputs=|--
  cos : Trigonometry  Operator=cos
  Out1 : Outport
  wires:
  Phase/1 -> Sum3/1
  Complex Exponential4/1 -> Gain1/1
  Sum3/1 -> Complex Exponential4/1  "Phase"
  Angle/1 -> cos/1
  Fm/1 -> Divide2/1
  cos/1 -> Divide2/2
  time/1 -> Product1/1
  Divide2/1 -> Product1/2
  Product1/1 -> Sum3/2
  Gain1/1 -> Product2/1
  Product2/1 -> Out1/1
  signal/1 -> Product2/2

== system multipath_fading1/path21 to path40, 20 paths/path31 to path40, 10 paths/path36 to path40, 5 paths/path36 ==
  note: initial phase
      | 0-2pi
      | uniformly
      | distributed
  note: incidence angle
      | 0-2pi
      | uniformity
      | distributed
  note: gain
      | 0-1uniformly distributed
  note: Fm_A
  Fm : Inport
  time : Inport  Port=2
  signal : Inport  Port=3
  Angle : Constant  Value=rand(1)*2*pi
  Complex Exponential4 : dspmathops/Complex Exponential
  Divide2 : Product  Inputs=**  OutScaling=2^-10
  Gain1 : Gain  Gain=rand(1)
  Phase : Constant  Value=rand(1)*2*pi
  Product1 : Product  RndMeth=Zero
  Product2 : Product  RndMeth=Zero
  Sum3 : Sum  Inputs=|--
  cos : Trigonometry  Operator=cos
  Out1 : Outport
  wires:
  Phase/1 -> Sum3/1
  Complex Exponential4/1 -> Gain1/1
  Sum3/1 -> Complex Exponential4/1  "Phase"
  Angle/1 -> cos/1
  Fm/1 -> Divide2/1
  cos/1 -> Divide2/2
  time/1 -> Product1/1
  Divide2/1 -> Product1/2
  Product1/1 -> Sum3/2
  Gain1/1 -> Product2/1
  Product2/1 -> Out1/1
  signal/1 -> Product2/2

== system multipath_fading1/path21 to path40, 20 paths/path31 to path40, 10 paths/path36 to path40, 5 paths/path37 ==
  note: initial phase
      | 0-2pi
      | uniformly
      | distributed
  note: incidence angle
      | 0-2pi
      | uniformity
      | distributed
  note: gain
      | 0-1uniformly distributed
  note: Fm_A
  Fm : Inport
  time : Inport  Port=2
  signal : Inport  Port=3
  Angle : Constant  Value=rand(1)*2*pi
  Complex Exponential4 : dspmathops/Complex Exponential
  Divide2 : Product  Inputs=**  OutScaling=2^-10
  Gain1 : Gain  Gain=rand(1)
  Phase : Constant  Value=rand(1)*2*pi
  Product1 : Product  RndMeth=Zero
  Product2 : Product  RndMeth=Zero
  Sum3 : Sum  Inputs=|--
  cos : Trigonometry  Operator=cos
  Out1 : Outport
  wires:
  Phase/1 -> Sum3/1
  Complex Exponential4/1 -> Gain1/1
  Sum3/1 -> Complex Exponential4/1  "Phase"
  Angle/1 -> cos/1
  Fm/1 -> Divide2/1
  cos/1 -> Divide2/2
  time/1 -> Product1/1
  Divide2/1 -> Product1/2
  Product1/1 -> Sum3/2
  Gain1/1 -> Product2/1
  Product2/1 -> Out1/1
  signal/1 -> Product2/2

== system multipath_fading1/path21 to path40, 20 paths/path31 to path40, 10 paths/path36 to path40, 5 paths/path38 ==
  note: initial phase
      | 0-2pi
      | uniformly
      | distributed
  note: incidence angle
      | 0-2pi
      | uniformity
      | distributed
  note: gain
      | 0-1uniformly distributed
  note: Fm_A
  Fm : Inport
  time : Inport  Port=2
  signal : Inport  Port=3
  Angle : Constant  Value=rand(1)*2*pi
  Complex Exponential4 : dspmathops/Complex Exponential
  Divide2 : Product  Inputs=**  OutScaling=2^-10
  Gain1 : Gain  Gain=rand(1)
  Phase : Constant  Value=rand(1)*2*pi
  Product1 : Product  RndMeth=Zero
  Product2 : Product  RndMeth=Zero
  Sum3 : Sum  Inputs=|--
  cos : Trigonometry  Operator=cos
  Out1 : Outport
  wires:
  Phase/1 -> Sum3/1
  Complex Exponential4/1 -> Gain1/1
  Sum3/1 -> Complex Exponential4/1  "Phase"
  Angle/1 -> cos/1
  Fm/1 -> Divide2/1
  cos/1 -> Divide2/2
  time/1 -> Product1/1
  Divide2/1 -> Product1/2
  Product1/1 -> Sum3/2
  Gain1/1 -> Product2/1
  Product2/1 -> Out1/1
  signal/1 -> Product2/2

== system multipath_fading1/path21 to path40, 20 paths/path31 to path40, 10 paths/path36 to path40, 5 paths/path39 ==
  note: initial phase
      | 0-2pi
      | uniformly
      | distributed
  note: incidence angle
      | 0-2pi
      | uniformity
      | distributed
  note: gain
      | 0-1uniformly distributed
  note: Fm_A
  Fm : Inport
  time : Inport  Port=2
  signal : Inport  Port=3
  Angle : Constant  Value=rand(1)*2*pi
  Complex Exponential4 : dspmathops/Complex Exponential
  Divide2 : Product  Inputs=**  OutScaling=2^-10
  Gain1 : Gain  Gain=rand(1)
  Phase : Constant  Value=rand(1)*2*pi
  Product1 : Product  RndMeth=Zero
  Product2 : Product  RndMeth=Zero
  Sum3 : Sum  Inputs=|--
  cos : Trigonometry  Operator=cos
  Out1 : Outport
  wires:
  Phase/1 -> Sum3/1
  Complex Exponential4/1 -> Gain1/1
  Sum3/1 -> Complex Exponential4/1  "Phase"
  Angle/1 -> cos/1
  Fm/1 -> Divide2/1
  cos/1 -> Divide2/2
  time/1 -> Product1/1
  Divide2/1 -> Product1/2
  Product1/1 -> Sum3/2
  Gain1/1 -> Product2/1
  Product2/1 -> Out1/1
  signal/1 -> Product2/2
